simulink model "Hardware_deploy_model"  (R2019a)
settings: Solver=FixedStepDiscrete  StartTime=0.0  StopTime=inf  RelTol=1e-3
model workspace (MAT data in the model file):
  actuatorCentres : struct (value not decoded)
  MCOS : class17 (value not decoded)
  MCOS : class17 (value not decoded)
  servoPins : struct (value not decoded)
undefined symbols (not defined in the file or in its folder): Aileron, DiscIntNeverNeededParam, Discrete, Elevator, Newton, Raphson, Time
libraries: simulink x13, arduinolib x11, ctrlSharedLib x3, aerolibtransform2 x3, dspsigops x2, sharedtransform x2, aerolibutil x1, simulink_extras x1
(part 2 of 2)

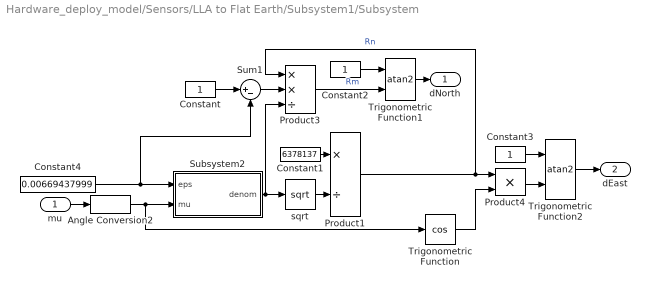
== system Hardware_deploy_model/Sensors/LLA to Flat Earth/Subsystem1/Subsystem ==
  mu : Inport
  Angle Conversion2 : aerolibtransform2/LLA to Flat Earth/Subsystem/Find Radian//Distance/Angle Conversion2  SystemSampleTime=-1
      settings: SourceProductName=Aerospace Blockset  SourceProductBaseCode=AE
  Constant : Constant  OutDataTypeStr=single
  Constant1 : Constant  Value=6378137  OutDataTypeStr=single
  Constant2 : Constant  OutDataTypeStr=single
  Constant3 : Constant  OutDataTypeStr=single
  Constant4 : Constant  Value=0.00669437999  OutDataTypeStr=single
  Product1 : Product  Inputs=*/  RndMeth=Zero
  Product3 : Product  Inputs=**/  OutDataTypeStr=single  RndMeth=Zero
  Product4 : Product  RndMeth=Zero
  Subsystem2 : Subsystem
  Sum1 : Sum  Inputs=|+-
  Trigonometric Function : Trigonometry  Operator=cos
  Trigonometric Function1 : Trigonometry  Operator=atan2
  Trigonometric Function2 : Trigonometry  Operator=atan2
  sqrt : Sqrt  AlgorithmType=Newton-Raphson  SaturateOnIntegerOverflow=on
  dNorth : Outport
  dEast : Outport  Port=2
  wires:
  Angle Conversion2/1 -> Subsystem2/2(mu), Trigonometric Function/1
  Constant/1 -> Sum1/1
  Trigonometric Function2/1 -> dEast/1
  Constant2/1 -> Trigonometric Function1/1
  Constant4/1 -> Sum1/2, Subsystem2/1(eps)
  sqrt/1 -> Product1/2
  Subsystem2/1(denom) -> Product3/3, sqrt/1
  Trigonometric Function/1 -> Product4/2
  Product1/1 -> Product3/1, Product4/1  "Rn"
  Trigonometric Function1/1 -> dNorth/1
  Product3/1 -> Trigonometric Function1/2  "Rm"
  Sum1/1 -> Product3/2
  Product4/1 -> Trigonometric Function2/2
  Constant1/1 -> Product1/1
  Constant3/1 -> Trigonometric Function2/1
  mu/1 -> Angle Conversion2/1

== system Hardware_deploy_model/Sensors/LLA to Flat Earth/LatLong wrap/Latitude Wrap 90/Wrap Angle 180 ==
  Angle : Inport
  Abs : Abs
  Bias : Bias  Bias=180
  Bias1 : Bias  Bias=-180
  Compare To Constant : simulink/Logic and Bit Operations/Compare To Constant  relop=>  const=180  OutDataTypeStr=boolean
  Constant2 : Constant  Value=360  OutDataTypeStr=single
  Math Function1 : Math  Operator=mod  SaturateOnIntegerOverflow=on
  Switch : Switch  Criteria=u2 ~= 0  Threshold=180
  Angle 180 : Outport
  wires:
  Compare To Constant/1 -> Switch/2
  Angle/1 -> Bias/1, Switch/3, Abs/1
  Abs/1 -> Compare To Constant/1
  Bias/1 -> Math Function1/1
  Constant2/1 -> Math Function1/2
  Math Function1/1 -> Bias1/1
  Bias1/1 -> Switch/1
  Switch/1 -> Angle 180/1

== system Hardware_deploy_model/Sensors/LLA to Flat Earth/LatLong wrap LL0/Latitude Wrap 90/Wrap Angle 180 ==
  Angle : Inport
  Abs : Abs
  Bias : Bias  Bias=180
  Bias1 : Bias  Bias=-180
  Compare To Constant : simulink/Logic and Bit Operations/Compare To Constant  relop=>  const=180  OutDataTypeStr=boolean
  Constant : Constant  Value=360  OutDataTypeStr=single
  Math Function1 : Math  Operator=mod  SaturateOnIntegerOverflow=on
  Switch : Switch  Criteria=u2 ~= 0  Threshold=180
  Angle 180 : Outport
  wires:
  Compare To Constant/1 -> Switch/2
  Angle/1 -> Bias/1, Switch/3, Abs/1
  Abs/1 -> Compare To Constant/1
  Bias/1 -> Math Function1/1
  Constant/1 -> Math Function1/2
  Math Function1/1 -> Bias1/1
  Bias1/1 -> Switch/1
  Switch/1 -> Angle 180/1

== system Hardware_deploy_model/Sensors/LLA to Flat Earth/Subsystem1/Subsystem/Subsystem2 ==
  eps : Inport
  mu : Inport  Port=2
  Constant : Constant  OutDataTypeStr=single
  Product1 : Product  Inputs=3  OutDataTypeStr=single  RndMeth=Zero
  Sum1 : Sum  Inputs=|+-
  Trigonometric Function1 : Trigonometry
  denom : Outport
  wires:
  Product1/1 -> Sum1/2
  Trigonometric Function1/1 -> Product1/2, Product1/3
  Constant/1 -> Sum1/1
  eps/1 -> Product1/1
  Sum1/1 -> denom/1
  mu/1 -> Trigonometric Function1/1
